simulink model "CukConverter"  (R2023b)
settings: Solver=VariableStepAuto  StartTime=0.0  StopTime=0.1  RelTol=1e-3
libraries: spsCurrentMeasurementLib x5, spsSeriesRLCBranchLib x5, spsVoltageMeasurementLib x2, spsDCVoltageSourceLib x1, spsDiodeLib x1, spsMosfetLib x1, sps_lib x1
settings Model: Creator=yagiz  LastModifiedBy=yagiz

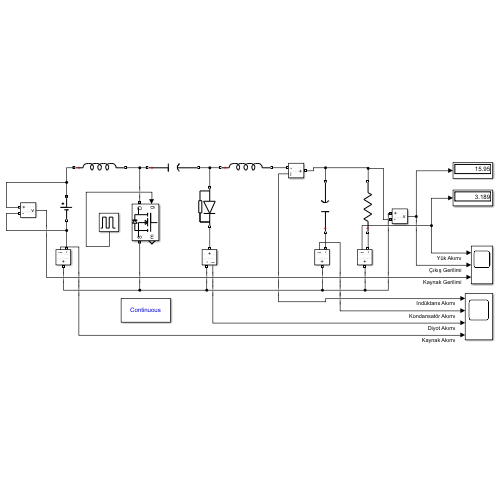
[thumbnail: Simulink's stored preview of the top-level diagram]
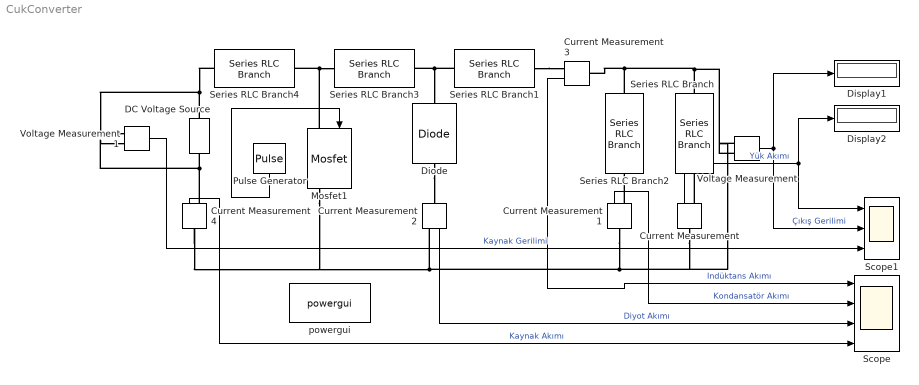
== system CukConverter ==
  Current Measurement{,1..4} (5 alike) : spsCurrentMeasurementLib/Current Measurement  PhasorSimulation=off  OutputType=Complex  PSBequivalent=0
  DC Voltage Source : spsDCVoltageSourceLib/DC Voltage Source  Amplitude=48  Measurements=None
  Diode : spsDiodeLib/Diode  Ron=0.001  Lon=0  Vf=0  IC=0  UseSnubber=0  Rs=500  Cs=250e-9  Measurements=off
  Display1 : Display
  Display2 : Display
  Mosfet1 : spsMosfetLib/Mosfet  Ron=0.04  Lon=0  Rd=0.00635  Vfd=1.2  IC=0  Rs=1e5  Cs=inf  Measurements=on
  Pulse Generator : DiscretePulseGenerator  PulseType=Time based  Period=1/40000  PulseWidth=25
  Scope : Scope  NumInputPorts=4
  Scope1 : Scope  NumInputPorts=3
  Series RLC Branch : spsSeriesRLCBranchLib/Series RLC Branch  LConnTagsString=__new0  RConnTagsString=__new0  BranchType=R  Resistance=5  Inductance=1e-3  SetiL0=off  InitialCurrent=0  Capacitance=1e-6  Setx0=off  InitialVoltage=0  Measurements=None
  Series RLC Branch1 : spsSeriesRLCBranchLib/Series RLC Branch  LConnTagsString=__new0  RConnTagsString=__new0  BranchType=L  Resistance=1  Inductance=5e-3  SetiL0=off  InitialCurrent=0  Capacitance=1e-6  Setx0=off  InitialVoltage=0  Measurements=None
  Series RLC Branch2 : spsSeriesRLCBranchLib/Series RLC Branch  LConnTagsString=__new0  RConnTagsString=__new0  BranchType=C  Resistance=1  Inductance=1e-3  SetiL0=off  InitialCurrent=0  Capacitance=100e-6  Setx0=off  InitialVoltage=0  Measurements=None
  Series RLC Branch3 : spsSeriesRLCBranchLib/Series RLC Branch  LConnTagsString=__new0  RConnTagsString=__new0  BranchType=C  Resistance=1  Inductance=1e-3  SetiL0=off  InitialCurrent=0  Capacitance=100e-6  Setx0=off  InitialVoltage=0  Measurements=None
  Series RLC Branch4 : spsSeriesRLCBranchLib/Series RLC Branch  LConnTagsString=__new0  RConnTagsString=__new0  BranchType=L  Resistance=1  Inductance=5e-3  SetiL0=off  InitialCurrent=0  Capacitance=1e-6  Setx0=off  InitialVoltage=0  Measurements=None
  Voltage Measurement : spsVoltageMeasurementLib/Voltage Measurement  PhasorSimulation=off  OutputType=Complex  PSBequivalent=0
  Voltage Measurement1 : spsVoltageMeasurementLib/Voltage Measurement  PhasorSimulation=off  OutputType=Complex  PSBequivalent=0
  powergui : sps_lib/powergui  Priority=1  SimulationMode=Continuous  SampleTime=5e-6  frequency=60  Iterations=50  frequencyindice=0  Pbase=100e6  ErrMax=1e-4  UnitsV=kV  UnitsW=MW  buscounter=0  FunctionMessages=off  echomessages=off  EnableUseOfTLC=off  CurrentSourceSwitches=off  DisableSnubberDevices=off  DisableRonSwitches=off  DisableVfSwitches=off  DisplayEquations=off  AutomaticDiscreteSolvers=off  SolverType=Tustin/Backward Euler (TBE)  Interpol=off  ExternalGateDelay=off  methode=off  Ts=100  x0status=blocks  SPID=on  SwTol=0  HookPort=off  NonlinearTolerance=1e-4  nMaxIteration=100  ContinueOnMaxIteration=off  RestoreLinks=warning  ResistiveCurrentMeasurement=off  Frange=[0:2:500]  Ylog=off  Xlog=on  ShowGrid=off  save=off  variable=ZData  structure=0  ZoomFFT=off  StartTime=0.0  cycles=1  DisplayStyle=1  fundamental=60  FreqAxis=off  MaxFrequency=1000  frequencyindicesteady=1  RmsSteady=1  display=off
  wires:
  Voltage Measurement/1 -> Display1/1, Scope1/2  "Çıkış Gerilimi"
  Current Measurement3/1 -> Scope/1  "Indüktans Akımı"
  Voltage Measurement1/1 -> Scope1/3  "Kaynak Gerilimi"
  Current Measurement4/1 -> Scope/4  "Kaynak Akımı"
  Current Measurement1/1 -> Scope/2  "Kondansatör Akımı"
  Current Measurement/1 -> Display2/1, Scope1/1  "Yük Akımı"
  Current Measurement2/1 -> Scope/3  "Diyot Akımı"
  Pulse Generator/1 -> Mosfet1/1
  connections:
  Current Measurement1/LConn1 -- Voltage Measurement/LConn1 -- Current Measurement/LConn1 -- Current Measurement4/LConn1 -- Mosfet1/RConn1 -- Current Measurement2/RConn1
  Series RLC Branch1/LConn1 -- Series RLC Branch3/RConn1 -- Diode/LConn1
  Series RLC Branch/RConn1 -- Current Measurement3/LConn1 -- Series RLC Branch2/RConn1 -- Voltage Measurement/LConn2
  DC Voltage Source/RConn1 -- Series RLC Branch4/LConn1 -- Voltage Measurement1/LConn1
  DC Voltage Source/LConn1 -- Current Measurement4/RConn1 -- Voltage Measurement1/LConn2
  Diode/RConn1 -- Current Measurement2/LConn1
  Current Measurement1/RConn1 -- Series RLC Branch2/LConn1
  Current Measurement/RConn1 -- Series RLC Branch/LConn1
  Series RLC Branch1/RConn1 -- Current Measurement3/RConn1
  Mosfet1/LConn1 -- Series RLC Branch4/RConn1 -- Series RLC Branch3/LConn1
